simulink model "threePhase_SPWM"  (R2022b)
settings: Solver=VariableStepAuto  StartTime=0.0  StopTime=0.1  RelTol=1e-3
libraries: simulink x3, hdlsllib x1, dspsrcs4 x1
settings Model: Creator=BAYINDIR  LastModifiedBy=BAYINDIR
settings OptimizationCC: BlockReduction=off  ConditionallyExecuteInputs=off

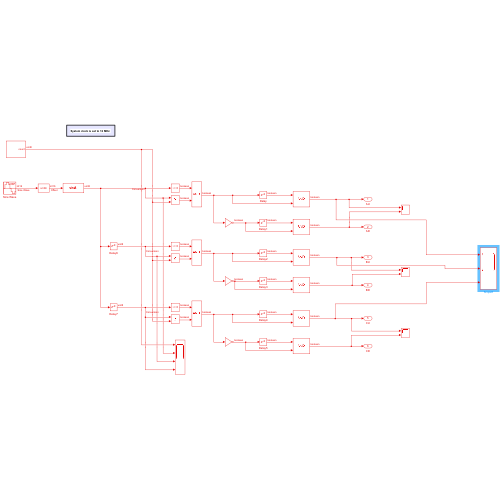
[thumbnail: Simulink's stored preview of the top-level diagram]
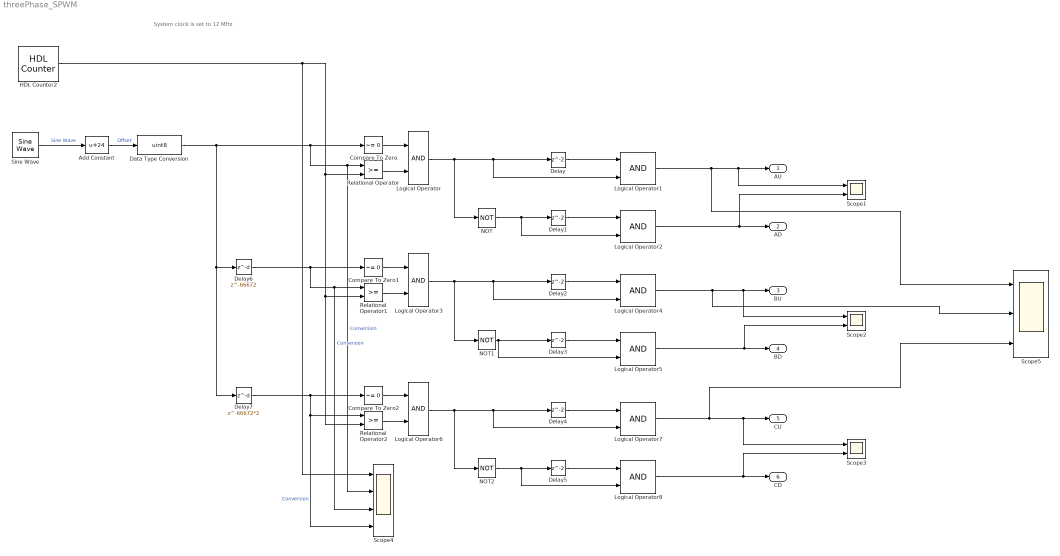
== system threePhase_SPWM ==
  note: System clock is set to 12 MHz
  Add Constant : Bias  Bias=24  SaturateOnIntegerOverflow=off
  Compare To Zero : simulink/Logic and Bit Operations/Compare To Zero  relop=~=  OutDataTypeStr=boolean
  Compare To Zero1 : simulink/Logic and Bit Operations/Compare To Zero  relop=~=  OutDataTypeStr=boolean
  Compare To Zero2 : simulink/Logic and Bit Operations/Compare To Zero  relop=~=  OutDataTypeStr=boolean
  Data Type Conversion : DataTypeConversion  OutMin=[0]  OutMax=[120]  OutDataTypeStr=uint8  SaturateOnIntegerOverflow=off  RndMeth=Floor
  Delay{,1..5} (6 alike) : Delay  InitialCondition=0  UseCircularBuffer=on
  Delay6 : Delay  DelayLength=66672  InitialCondition=0  UseCircularBuffer=on
  Delay7 : Delay  DelayLength=66672*2  InitialCondition=0  UseCircularBuffer=on
  HDL Counter2 : hdlsllib/Sources/HDL Counter  CountType=Count limited  CountInit=0  CountStep=1  CountMax=60  CountFromType=Initial value  CountFrom=0  CountResetPort=off  CountLoadPort=off  CountEnbPort=off  CountDirPort=off  CountHitOutputPort=off  CountDataType=Unsigned  CountWordLen=8  CountFracLen=0  CountSampTime=1/12e6
  Logical Operator{,1..8} (9 alike) : Logic  AllPortsSameDT=off  OutDataTypeStr=boolean
  NOT : Logic  Operator=NOT  IconShape=distinctive  AllPortsSameDT=off  OutDataTypeStr=boolean
  NOT1 : Logic  Operator=NOT  IconShape=distinctive  AllPortsSameDT=off  OutDataTypeStr=boolean
  NOT2 : Logic  Operator=NOT  IconShape=distinctive  AllPortsSameDT=off  OutDataTypeStr=boolean
  Relational Operator : RelationalOperator  OutDataTypeStr=boolean  RndMeth=Simplest  InputSameDT=off
  Relational Operator1 : RelationalOperator  OutDataTypeStr=boolean  RndMeth=Simplest  InputSameDT=off
  Relational Operator2 : RelationalOperator  OutDataTypeStr=boolean  RndMeth=Simplest  InputSameDT=off
  Scope1 : Scope  NumInputPorts=2
  Scope2 : Scope  NumInputPorts=2
  Scope3 : Scope  NumInputPorts=2
  Scope4 : Scope  NumInputPorts=4
  Scope5 : Scope  NumInputPorts=3
  Sine Wave : dspsrcs4/Sine Wave  Amplitude=24  Frequency=60  Phase=0  SampleMode=Discrete  OutComplex=Real  CompMethod=Table lookup  TableSize=Memory  SampleTime=1/12e6  SamplesPerFrame=1  ResetState=Restart at time zero  OutputFrames=off  dataType=Fixed-point  wordLen=16  udDataType=sfix(16)  fracBitsMode=User-defined  numFracBits=0  OutDataTypeStr=fixdt(1,16,0)  LastOutDataTypeStr=fixdt(1,16,0)
  AU : Outport  VectorParamsAs1DForOutWhenUnconnected=off
  AD : Outport  Port=2  VectorParamsAs1DForOutWhenUnconnected=off
  BU : Outport  Port=3  VectorParamsAs1DForOutWhenUnconnected=off
  BD : Outport  Port=4  VectorParamsAs1DForOutWhenUnconnected=off
  CU : Outport  Port=5  VectorParamsAs1DForOutWhenUnconnected=off
  CD : Outport  Port=6  VectorParamsAs1DForOutWhenUnconnected=off
  wires:
  Logical Operator2/1 -> Scope1/2, AD/1
  NOT/1 -> Logical Operator2/2, Delay1/1
  Data Type Conversion/1 -> Scope4/2, Relational Operator/1, Compare To Zero/1, Delay7/1, Delay6/1  "Conversion"
  Delay1/1 -> Logical Operator2/1
  Logical Operator/1 -> Logical Operator1/2, Delay/1, NOT/1
  Add Constant/1 -> Data Type Conversion/1  "Offset"
  Delay/1 -> Logical Operator1/1
  Compare To Zero/1 -> Logical Operator/1
  Relational Operator/1 -> Logical Operator/2
  Logical Operator1/1 -> Scope5/1, Scope1/1, AU/1
  Sine Wave/1 -> Add Constant/1  "Sine Wave"
  Delay3/1 -> Logical Operator5/1
  Logical Operator3/1 -> Logical Operator4/2, Delay2/1, NOT1/1
  Logical Operator4/1 -> Scope5/2, BU/1, Scope2/1
  Delay2/1 -> Logical Operator4/1
  Compare To Zero1/1 -> Logical Operator3/1
  Logical Operator5/1 -> Scope2/2, BD/1
  Delay6/1 -> Scope4/3, Relational Operator1/1, Compare To Zero1/1  "Conversion"
  Relational Operator1/1 -> Logical Operator3/2
  NOT1/1 -> Logical Operator5/2, Delay3/1
  Delay5/1 -> Logical Operator8/1
  Logical Operator6/1 -> Logical Operator7/2, Delay4/1, NOT2/1
  Logical Operator7/1 -> Scope5/3, CU/1, Scope3/1
  Delay4/1 -> Logical Operator7/1
  Compare To Zero2/1 -> Logical Operator6/1
  Logical Operator8/1 -> Scope3/2, CD/1
  Delay7/1 -> Relational Operator2/1, Scope4/4, Compare To Zero2/1  "Conversion"
  Relational Operator2/1 -> Logical Operator6/2
  NOT2/1 -> Logical Operator8/2, Delay5/1
  HDL Counter2/1 -> Scope4/1, Relational Operator2/2, Relational Operator1/2, Relational Operator/2
